simulink model "neuronchainv4"  (Simulink 7.6)
settings: Solver=ode45  StartTime=0.0  StopTime=10.0  RelTol=1e-3
values from neighbouring files (symbols this model uses):
  alpha = 0.8    [excneuroninit.m]
  beta = 0.05    [excneuroninit.m]
  inittime = 0.1    [excneuroninit.m]
  sigslopef = 1    [excneuroninit.m]
  sigslopei = 3    [excneuroninit.m]
  tau_s = 5    [excneuroninit.m]
libraries: simulink x480, neuronpoolibv3 x3
(part 1 of 17)
settings Model: Creator=root  LastModifiedBy=root

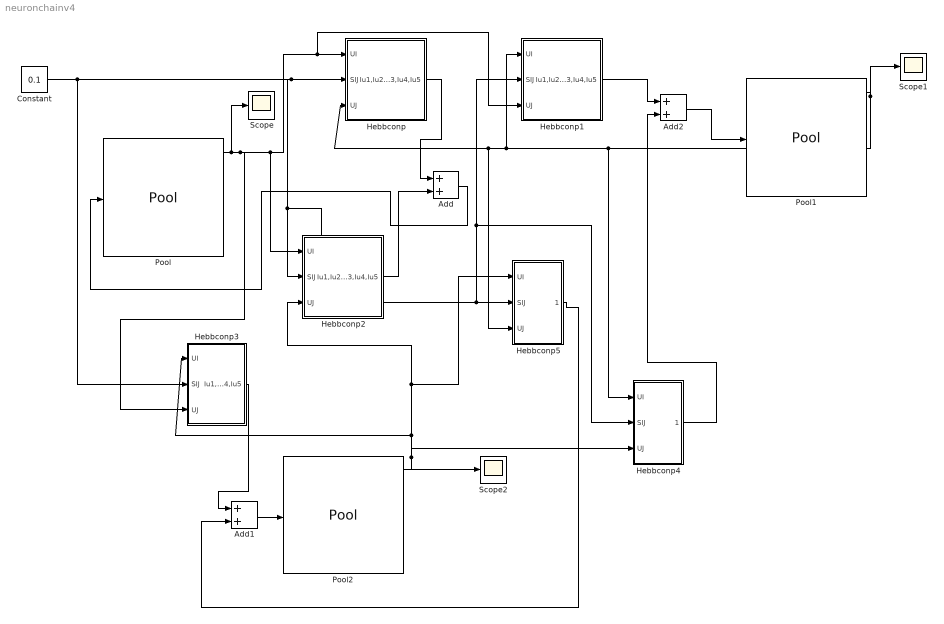
== system neuronchainv4 ==
  Add : Sum
  Add1 : Sum
  Add2 : Sum
  Constant : Constant  Value=0.1
  Hebbconp : Subsystem
  Hebbconp1 : Subsystem
  Hebbconp2 : Subsystem
  Hebbconp3 : Subsystem
  Hebbconp4 : Subsystem
  Hebbconp5 : Subsystem
  Pool : neuronpoolibv3/Pool  SystemSampleTime=-1
  Pool1 : neuronpoolibv3/Pool  SystemSampleTime=-1
  Pool2 : neuronpoolibv3/Pool  SystemSampleTime=-1
  Scope : Scope
  Scope1 : Scope
  Scope2 : Scope
      settings: SaveName=ScopeData2
  wires:
  Pool/1 -> Hebbconp/1(UI), Hebbconp1/3(UJ), Hebbconp2/1(UI), Hebbconp3/3(UJ), Scope/1
  Pool1/1 -> Hebbconp/3(UJ), Hebbconp5/3(UJ), Hebbconp1/1(UI), Hebbconp4/1(UI), Scope1/1
  Pool2/1 -> Hebbconp2/3(UJ), Hebbconp5/1(UI), Hebbconp3/1(UI), Scope2/1, Hebbconp4/3(UJ)
  Hebbconp2/1(Iu1,Iu2,Iu3,Iu4,Iu5) -> Add/2
  Hebbconp/1(Iu1,Iu2,Iu3,Iu4,Iu5) -> Add/1
  Add/1 -> Pool/1
  Hebbconp5/1(Iu1,Iu2,Iu3,Iu4,Iu5) -> Add1/2
  Hebbconp3/1(Iu1,Iu2,Iu3,Iu4,Iu5) -> Add1/1
  Add1/1 -> Pool2/1
  Hebbconp4/1(Iu1,Iu2,Iu3,Iu4,Iu5) -> Add2/2
  Hebbconp1/1(Iu1,Iu2,Iu3,Iu4,Iu5) -> Add2/1
  Add2/1 -> Pool1/1
  Constant/1 -> Hebbconp/2(SIJ), Hebbconp1/2(SIJ), Hebbconp4/2(SIJ), Hebbconp5/2(SIJ), Hebbconp2/2(SIJ), Hebbconp3/2(SIJ)

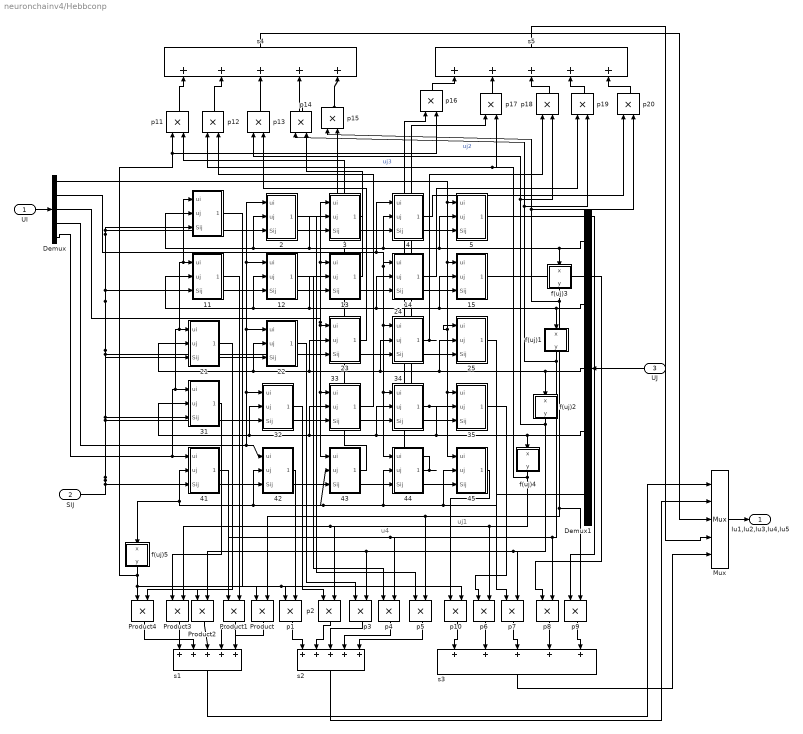
== system neuronchainv4/Hebbconp ==
  note: uj1
  note: u4
  UI : Inport
  SIJ : Inport  Port=2
  UJ : Inport  Port=3
  " " : Subsystem
  " 2" : Subsystem
  11 : Subsystem
  12 : Subsystem
  13 : Subsystem
  14 : Subsystem
  15 : Subsystem
  21 : Subsystem
  22 : Subsystem
  23 : Subsystem
  24 : Subsystem
  25 : Subsystem
  3 : Subsystem
  31 : Subsystem
  32 : Subsystem
  33 : Subsystem
  34 : Subsystem
  35 : Subsystem
  4 : Subsystem
  41 : Subsystem
  42 : Subsystem
  43 : Subsystem
  44 : Subsystem
  45 : Subsystem
  5 : Subsystem
  Demux : Demux  Outputs=5
  Demux1 : Demux  Outputs=5
  Mux : Mux  Inputs=5
  Product{,1..4} (5 alike) : Product  RndMeth=Zero
  f(uj)1 : Subsystem  TreatAsAtomicUnit=on  mask{slope=sigslopef, offset=0.5}
      mask help: Created by Han, Cheol
      mask Display: plot([10 15 20 25 30 35 40 45 50], [0 0.01 0.1 0.2 0.5 0.8 0.9 0.99 1])
  f(uj)2 : Subsystem  TreatAsAtomicUnit=on  mask{slope=sigslopef, offset=0.5}
      mask help: Created by Han, Cheol
      mask Display: plot([10 15 20 25 30 35 40 45 50], [0 0.01 0.1 0.2 0.5 0.8 0.9 0.99 1])
  f(uj)3 : Subsystem  TreatAsAtomicUnit=on  mask{slope=sigslopef, offset=0.5}
      mask help: Created by Han, Cheol
      mask Display: plot([10 15 20 25 30 35 40 45 50], [0 0.01 0.1 0.2 0.5 0.8 0.9 0.99 1])
  f(uj)4 : Subsystem  TreatAsAtomicUnit=on  mask{slope=sigslopef, offset=0.5}
      mask help: Created by Han, Cheol
      mask Display: plot([10 15 20 25 30 35 40 45 50], [0 0.01 0.1 0.2 0.5 0.8 0.9 0.99 1])
  f(uj)5 : Subsystem  TreatAsAtomicUnit=on  mask{slope=sigslopef, offset=0.5}
      mask help: Created by Han, Cheol
      mask Display: plot([10 15 20 25 30 35 40 45 50], [0 0.01 0.1 0.2 0.5 0.8 0.9 0.99 1])
  p{1..20} (20 alike) : Product  RndMeth=Zero
  s{1..5} (5 alike) : Sum  Inputs=+++++
  Iu1,Iu2,Iu3,Iu4,Iu5 : Outport
  wires:
  Demux/1 -> 15/1(ui), 45/1(ui), 35/1(ui), 25/1(ui), 5/1(ui)
  Demux/2 -> 4/1(ui), 44/1(ui), 34/1(ui), 24/1(ui), 14/1(ui)
  Demux/3 -> 43/1(ui), 33/1(ui), 23/1(ui), 13/1(ui), 3/1(ui)
  Demux/4 -> 42/1(ui), 32/1(ui), 22/1(ui), 12/1(ui), " 2"/1(ui)
  Demux/5 -> 41/1(ui), 31/1(ui), 21/1(ui), 11/1(ui), " "/1(ui)
  Demux1/1 -> " "/2(uj), " 2"/2(uj), 3/2(uj), 4/2(uj), 5/2(uj), f(uj)3/1(x)
  Demux1/2 -> 11/2(uj), 12/2(uj), 13/2(uj), 14/2(uj), 15/2(uj), f(uj)1/1(x)
  Demux1/3 -> 25/2(uj), 21/2(uj), 22/2(uj), 23/2(uj), 24/2(uj), f(uj)2/1(x)
  Demux1/4 -> 31/2(uj), 32/2(uj), 33/2(uj), 34/2(uj), 35/2(uj), f(uj)4/1(x)
  Demux1/5 -> 42/2(uj), 41/2(uj), f(uj)5/1(x), 43/2(uj), 44/2(uj), 45/2(uj)
  " "/1(Out1) -> Product/1
  11/1(Out1) -> Product1/2
  41/1(Out1) -> Product4/2
  21/1(Out1) -> Product2/1
  31/1(Out1) -> Product3/1
  f(uj)3/1(y) -> Product/2, p5/2, p9/2, p15/1, p20/2
  f(uj)1/1(y) -> Product1/1, p4/2, p8/2, p14/1, p19/2  "uj2"
  f(uj)2/1(y) -> Product2/2, p3/2, p7/2, p13/1, p18/2  "uj3"
  f(uj)4/1(y) -> Product3/2, p2/2, p6/2, p17/2, p12/1
  " 2"/1(Out1) -> p5/1
  12/1(Out1) -> p4/1
  22/1(Out1) -> p3/1
  32/1(Out1) -> p2/1
  42/1(Out1) -> p1/2
  f(uj)5/1(y) -> Product4/1, p1/1, p10/2, p11/1, p16/2
  5/1(Out1) -> p9/1
  15/1(Out1) -> p8/1
  25/1(Out1) -> p7/1
  35/1(Out1) -> p6/1
  45/1(Out1) -> p10/1
  3/1(Out1) -> p15/2
  13/1(Out1) -> p14/2
  23/1(Out1) -> p13/2
  33/1(Out1) -> p12/2
  43/1(Out1) -> p11/2
  p15/1 -> s4/5
  p11/1 -> s4/1
  p12/1 -> s4/2
  p13/1 -> s4/3
  p14/1 -> s4/4
  UI/1 -> Demux/1
  4/1(Out1) -> p20/1
  SIJ/1 -> 41/3(Sij), 21/3(Sij), 11/3(Sij), " "/3(Sij), " 2"/3(Sij), 3/3(Sij), 4/3(Sij), 5/3(Sij), 13/3(Sij), 14/3(Sij), 15/3(Sij), 12/3(Sij), 22/3(Sij), 23/3(Sij), 24/3(Sij), 25/3(Sij), 31/3(Sij), 33/3(Sij), 34/3(Sij), 35/3(Sij), 32/3(Sij), 42/3(Sij), 43/3(Sij), 44/3(Sij), 45/3(Sij)
  14/1(Out1) -> p19/1
  24/1(Out1) -> p18/1
  UJ/1 -> Demux1/1
  34/1(Out1) -> p17/1
  44/1(Out1) -> p16/1
  Product/1 -> s1/5
  Product1/1 -> s1/4
  Product2/1 -> s1/3
  Product3/1 -> s1/2
  Product4/1 -> s1/1
  p1/1 -> s2/1
  p10/1 -> s3/1
  p2/1 -> s2/2
  p3/1 -> s2/3
  p4/1 -> s2/4
  p5/1 -> s2/5
  p6/1 -> s3/2
  p7/1 -> s3/3
  p8/1 -> s3/4
  p9/1 -> s3/5
  p16/1 -> s5/1
  p17/1 -> s5/2
  p18/1 -> s5/3
  p19/1 -> s5/4
  p20/1 -> s5/5
  s4/1 -> Mux/3
  s1/1 -> Mux/1
  s2/1 -> Mux/2
  s3/1 -> Mux/5
  s5/1 -> Mux/4
  Mux/1 -> Iu1,Iu2,Iu3,Iu4,Iu5/1

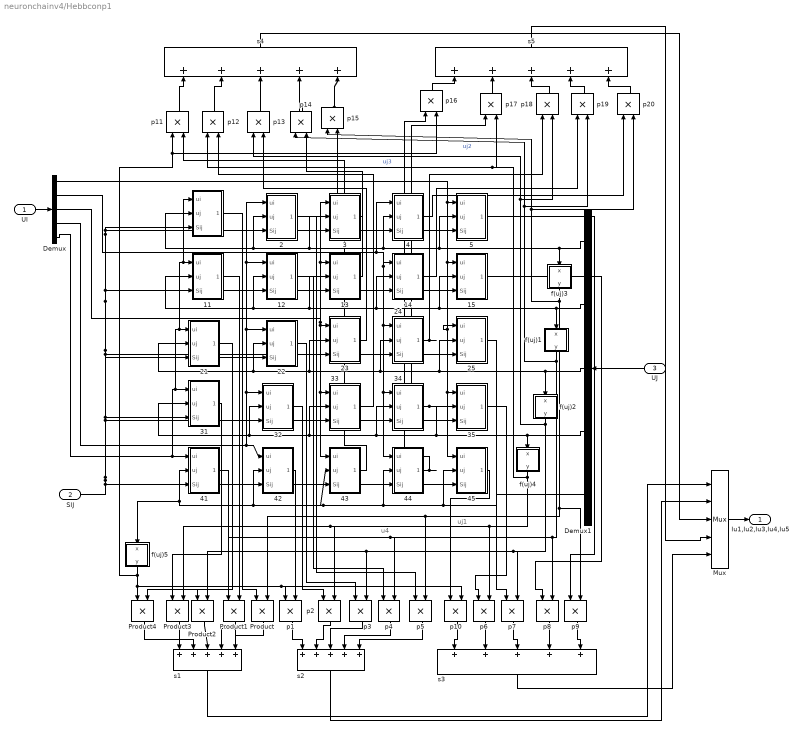
== system neuronchainv4/Hebbconp1 ==
  note: uj1
  note: u4
  UI : Inport
  SIJ : Inport  Port=2
  UJ : Inport  Port=3
  " " : Subsystem
  " 2" : Subsystem
  11 : Subsystem
  12 : Subsystem
  13 : Subsystem
  14 : Subsystem
  15 : Subsystem
  21 : Subsystem
  22 : Subsystem
  23 : Subsystem
  24 : Subsystem
  25 : Subsystem
  3 : Subsystem
  31 : Subsystem
  32 : Subsystem
  33 : Subsystem
  34 : Subsystem
  35 : Subsystem
  4 : Subsystem
  41 : Subsystem
  42 : Subsystem
  43 : Subsystem
  44 : Subsystem
  45 : Subsystem
  5 : Subsystem
  Demux : Demux  Outputs=5
  Demux1 : Demux  Outputs=5
  Mux : Mux  Inputs=5
  Product{,1..4} (5 alike) : Product  RndMeth=Zero
  f(uj)1 : Subsystem  TreatAsAtomicUnit=on  mask{slope=sigslopef, offset=0.5}
      mask help: Created by Han, Cheol
      mask Display: plot([10 15 20 25 30 35 40 45 50], [0 0.01 0.1 0.2 0.5 0.8 0.9 0.99 1])
  f(uj)2 : Subsystem  TreatAsAtomicUnit=on  mask{slope=sigslopef, offset=0.5}
      mask help: Created by Han, Cheol
      mask Display: plot([10 15 20 25 30 35 40 45 50], [0 0.01 0.1 0.2 0.5 0.8 0.9 0.99 1])
  f(uj)3 : Subsystem  TreatAsAtomicUnit=on  mask{slope=sigslopef, offset=0.5}
      mask help: Created by Han, Cheol
      mask Display: plot([10 15 20 25 30 35 40 45 50], [0 0.01 0.1 0.2 0.5 0.8 0.9 0.99 1])
  f(uj)4 : Subsystem  TreatAsAtomicUnit=on  mask{slope=sigslopef, offset=0.5}
      mask help: Created by Han, Cheol
      mask Display: plot([10 15 20 25 30 35 40 45 50], [0 0.01 0.1 0.2 0.5 0.8 0.9 0.99 1])
  f(uj)5 : Subsystem  TreatAsAtomicUnit=on  mask{slope=sigslopef, offset=0.5}
      mask help: Created by Han, Cheol
      mask Display: plot([10 15 20 25 30 35 40 45 50], [0 0.01 0.1 0.2 0.5 0.8 0.9 0.99 1])
  p{1..20} (20 alike) : Product  RndMeth=Zero
  s{1..5} (5 alike) : Sum  Inputs=+++++
  Iu1,Iu2,Iu3,Iu4,Iu5 : Outport
  wires:
  Demux/1 -> 15/1(ui), 45/1(ui), 35/1(ui), 25/1(ui), 5/1(ui)
  Demux/2 -> 4/1(ui), 44/1(ui), 34/1(ui), 24/1(ui), 14/1(ui)
  Demux/3 -> 43/1(ui), 33/1(ui), 23/1(ui), 13/1(ui), 3/1(ui)
  Demux/4 -> 42/1(ui), 32/1(ui), 22/1(ui), 12/1(ui), " 2"/1(ui)
  Demux/5 -> 41/1(ui), 31/1(ui), 21/1(ui), 11/1(ui), " "/1(ui)
  Demux1/1 -> " "/2(uj), " 2"/2(uj), 3/2(uj), 4/2(uj), 5/2(uj), f(uj)3/1(x)
  Demux1/2 -> 11/2(uj), 12/2(uj), 13/2(uj), 14/2(uj), 15/2(uj), f(uj)1/1(x)
  Demux1/3 -> 25/2(uj), 21/2(uj), 22/2(uj), 23/2(uj), 24/2(uj), f(uj)2/1(x)
  Demux1/4 -> 31/2(uj), 32/2(uj), 33/2(uj), 34/2(uj), 35/2(uj), f(uj)4/1(x)
  Demux1/5 -> 42/2(uj), 41/2(uj), f(uj)5/1(x), 43/2(uj), 44/2(uj), 45/2(uj)
  " "/1(Out1) -> Product/1
  11/1(Out1) -> Product1/2
  41/1(Out1) -> Product4/2
  21/1(Out1) -> Product2/1
  31/1(Out1) -> Product3/1
  f(uj)3/1(y) -> Product/2, p5/2, p9/2, p15/1, p20/2
  f(uj)1/1(y) -> Product1/1, p4/2, p8/2, p14/1, p19/2  "uj2"
  f(uj)2/1(y) -> Product2/2, p3/2, p7/2, p13/1, p18/2  "uj3"
  f(uj)4/1(y) -> Product3/2, p2/2, p6/2, p17/2, p12/1
  " 2"/1(Out1) -> p5/1
  12/1(Out1) -> p4/1
  22/1(Out1) -> p3/1
  32/1(Out1) -> p2/1
  42/1(Out1) -> p1/2
  f(uj)5/1(y) -> Product4/1, p1/1, p10/2, p11/1, p16/2
  5/1(Out1) -> p9/1
  15/1(Out1) -> p8/1
  25/1(Out1) -> p7/1
  35/1(Out1) -> p6/1
  45/1(Out1) -> p10/1
  3/1(Out1) -> p15/2
  13/1(Out1) -> p14/2
  23/1(Out1) -> p13/2
  33/1(Out1) -> p12/2
  43/1(Out1) -> p11/2
  p15/1 -> s4/5
  p11/1 -> s4/1
  p12/1 -> s4/2
  p13/1 -> s4/3
  p14/1 -> s4/4
  UI/1 -> Demux/1
  4/1(Out1) -> p20/1
  SIJ/1 -> 41/3(Sij), 21/3(Sij), 11/3(Sij), " "/3(Sij), " 2"/3(Sij), 3/3(Sij), 4/3(Sij), 5/3(Sij), 13/3(Sij), 14/3(Sij), 15/3(Sij), 12/3(Sij), 22/3(Sij), 23/3(Sij), 24/3(Sij), 25/3(Sij), 31/3(Sij), 33/3(Sij), 34/3(Sij), 35/3(Sij), 32/3(Sij), 42/3(Sij), 43/3(Sij), 44/3(Sij), 45/3(Sij)
  14/1(Out1) -> p19/1
  24/1(Out1) -> p18/1
  UJ/1 -> Demux1/1
  34/1(Out1) -> p17/1
  44/1(Out1) -> p16/1
  Product/1 -> s1/5
  Product1/1 -> s1/4
  Product2/1 -> s1/3
  Product3/1 -> s1/2
  Product4/1 -> s1/1
  p1/1 -> s2/1
  p10/1 -> s3/1
  p2/1 -> s2/2
  p3/1 -> s2/3
  p4/1 -> s2/4
  p5/1 -> s2/5
  p6/1 -> s3/2
  p7/1 -> s3/3
  p8/1 -> s3/4
  p9/1 -> s3/5
  p16/1 -> s5/1
  p17/1 -> s5/2
  p18/1 -> s5/3
  p19/1 -> s5/4
  p20/1 -> s5/5
  s4/1 -> Mux/3
  s1/1 -> Mux/1
  s2/1 -> Mux/2
  s3/1 -> Mux/5
  s5/1 -> Mux/4
  Mux/1 -> Iu1,Iu2,Iu3,Iu4,Iu5/1

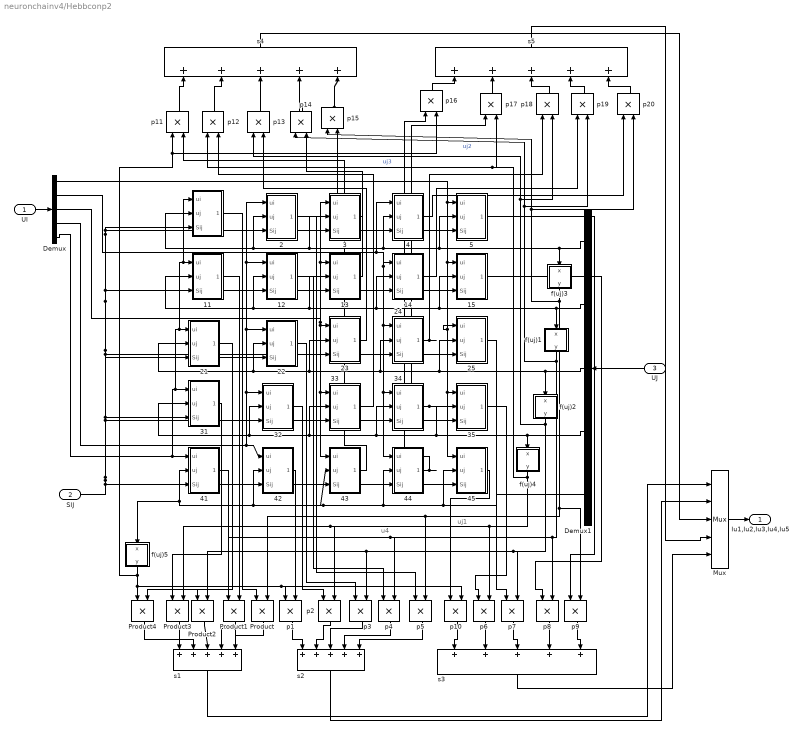
== system neuronchainv4/Hebbconp2 ==
  note: uj1
  note: u4
  UI : Inport
  SIJ : Inport  Port=2
  UJ : Inport  Port=3
  " " : Subsystem
  " 2" : Subsystem
  11 : Subsystem
  12 : Subsystem
  13 : Subsystem
  14 : Subsystem
  15 : Subsystem
  21 : Subsystem
  22 : Subsystem
  23 : Subsystem
  24 : Subsystem
  25 : Subsystem
  3 : Subsystem
  31 : Subsystem
  32 : Subsystem
  33 : Subsystem
  34 : Subsystem
  35 : Subsystem
  4 : Subsystem
  41 : Subsystem
  42 : Subsystem
  43 : Subsystem
  44 : Subsystem
  45 : Subsystem
  5 : Subsystem
  Demux : Demux  Outputs=5
  Demux1 : Demux  Outputs=5
  Mux : Mux  Inputs=5
  Product{,1..4} (5 alike) : Product  RndMeth=Zero
  f(uj)1 : Subsystem  TreatAsAtomicUnit=on  mask{slope=sigslopef, offset=0.5}
      mask help: Created by Han, Cheol
      mask Display: plot([10 15 20 25 30 35 40 45 50], [0 0.01 0.1 0.2 0.5 0.8 0.9 0.99 1])
  f(uj)2 : Subsystem  TreatAsAtomicUnit=on  mask{slope=sigslopef, offset=0.5}
      mask help: Created by Han, Cheol
      mask Display: plot([10 15 20 25 30 35 40 45 50], [0 0.01 0.1 0.2 0.5 0.8 0.9 0.99 1])
  f(uj)3 : Subsystem  TreatAsAtomicUnit=on  mask{slope=sigslopef, offset=0.5}
      mask help: Created by Han, Cheol
      mask Display: plot([10 15 20 25 30 35 40 45 50], [0 0.01 0.1 0.2 0.5 0.8 0.9 0.99 1])
  f(uj)4 : Subsystem  TreatAsAtomicUnit=on  mask{slope=sigslopef, offset=0.5}
      mask help: Created by Han, Cheol
      mask Display: plot([10 15 20 25 30 35 40 45 50], [0 0.01 0.1 0.2 0.5 0.8 0.9 0.99 1])
  f(uj)5 : Subsystem  TreatAsAtomicUnit=on  mask{slope=sigslopef, offset=0.5}
      mask help: Created by Han, Cheol
      mask Display: plot([10 15 20 25 30 35 40 45 50], [0 0.01 0.1 0.2 0.5 0.8 0.9 0.99 1])
  p{1..20} (20 alike) : Product  RndMeth=Zero
  s{1..5} (5 alike) : Sum  Inputs=+++++
  Iu1,Iu2,Iu3,Iu4,Iu5 : Outport
  wires:
  Demux/1 -> 15/1(ui), 45/1(ui), 35/1(ui), 25/1(ui), 5/1(ui)
  Demux/2 -> 4/1(ui), 44/1(ui), 34/1(ui), 24/1(ui), 14/1(ui)
  Demux/3 -> 43/1(ui), 33/1(ui), 23/1(ui), 13/1(ui), 3/1(ui)
  Demux/4 -> 42/1(ui), 32/1(ui), 22/1(ui), 12/1(ui), " 2"/1(ui)
  Demux/5 -> 41/1(ui), 31/1(ui), 21/1(ui), 11/1(ui), " "/1(ui)
  Demux1/1 -> " "/2(uj), " 2"/2(uj), 3/2(uj), 4/2(uj), 5/2(uj), f(uj)3/1(x)
  Demux1/2 -> 11/2(uj), 12/2(uj), 13/2(uj), 14/2(uj), 15/2(uj), f(uj)1/1(x)
  Demux1/3 -> 25/2(uj), 21/2(uj), 22/2(uj), 23/2(uj), 24/2(uj), f(uj)2/1(x)
  Demux1/4 -> 31/2(uj), 32/2(uj), 33/2(uj), 34/2(uj), 35/2(uj), f(uj)4/1(x)
  Demux1/5 -> 42/2(uj), 41/2(uj), f(uj)5/1(x), 43/2(uj), 44/2(uj), 45/2(uj)
  " "/1(Out1) -> Product/1
  11/1(Out1) -> Product1/2
  41/1(Out1) -> Product4/2
  21/1(Out1) -> Product2/1
  31/1(Out1) -> Product3/1
  f(uj)3/1(y) -> Product/2, p5/2, p9/2, p15/1, p20/2
  f(uj)1/1(y) -> Product1/1, p4/2, p8/2, p14/1, p19/2  "uj2"
  f(uj)2/1(y) -> Product2/2, p3/2, p7/2, p13/1, p18/2  "uj3"
  f(uj)4/1(y) -> Product3/2, p2/2, p6/2, p17/2, p12/1
  " 2"/1(Out1) -> p5/1
  12/1(Out1) -> p4/1
  22/1(Out1) -> p3/1
  32/1(Out1) -> p2/1
  42/1(Out1) -> p1/2
  f(uj)5/1(y) -> Product4/1, p1/1, p10/2, p11/1, p16/2
  5/1(Out1) -> p9/1
  15/1(Out1) -> p8/1
  25/1(Out1) -> p7/1
  35/1(Out1) -> p6/1
  45/1(Out1) -> p10/1
  3/1(Out1) -> p15/2
  13/1(Out1) -> p14/2
  23/1(Out1) -> p13/2
  33/1(Out1) -> p12/2
  43/1(Out1) -> p11/2
  p15/1 -> s4/5
  p11/1 -> s4/1
  p12/1 -> s4/2
  p13/1 -> s4/3
  p14/1 -> s4/4
  UI/1 -> Demux/1
  4/1(Out1) -> p20/1
  SIJ/1 -> 41/3(Sij), 21/3(Sij), 11/3(Sij), " "/3(Sij), " 2"/3(Sij), 3/3(Sij), 4/3(Sij), 5/3(Sij), 13/3(Sij), 14/3(Sij), 15/3(Sij), 12/3(Sij), 22/3(Sij), 23/3(Sij), 24/3(Sij), 25/3(Sij), 31/3(Sij), 33/3(Sij), 34/3(Sij), 35/3(Sij), 32/3(Sij), 42/3(Sij), 43/3(Sij), 44/3(Sij), 45/3(Sij)
  14/1(Out1) -> p19/1
  24/1(Out1) -> p18/1
  UJ/1 -> Demux1/1
  34/1(Out1) -> p17/1
  44/1(Out1) -> p16/1
  Product/1 -> s1/5
  Product1/1 -> s1/4
  Product2/1 -> s1/3
  Product3/1 -> s1/2
  Product4/1 -> s1/1
  p1/1 -> s2/1
  p10/1 -> s3/1
  p2/1 -> s2/2
  p3/1 -> s2/3
  p4/1 -> s2/4
  p5/1 -> s2/5
  p6/1 -> s3/2
  p7/1 -> s3/3
  p8/1 -> s3/4
  p9/1 -> s3/5
  p16/1 -> s5/1
  p17/1 -> s5/2
  p18/1 -> s5/3
  p19/1 -> s5/4
  p20/1 -> s5/5
  s4/1 -> Mux/3
  s1/1 -> Mux/1
  s2/1 -> Mux/2
  s3/1 -> Mux/5
  s5/1 -> Mux/4
  Mux/1 -> Iu1,Iu2,Iu3,Iu4,Iu5/1

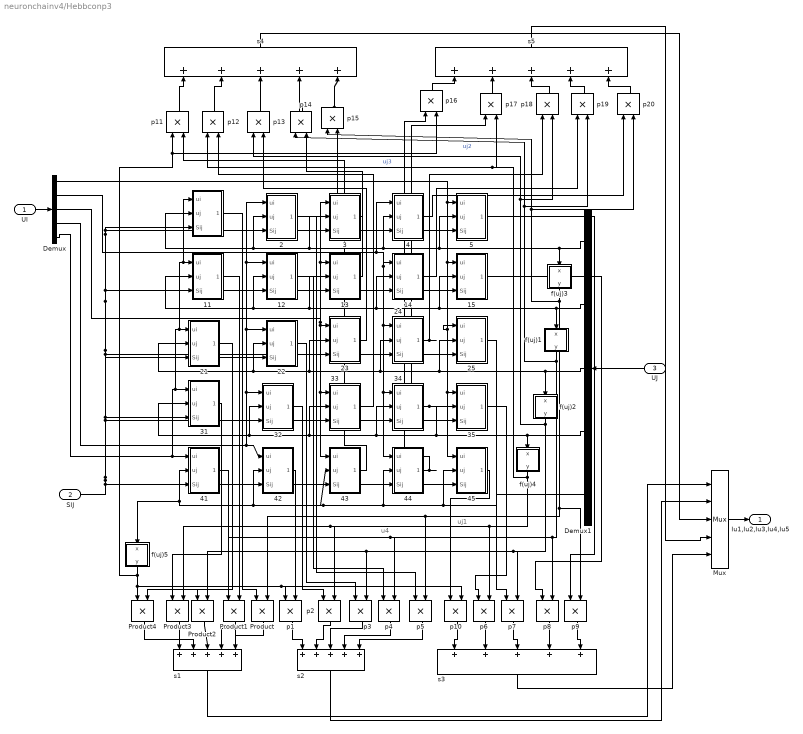
== system neuronchainv4/Hebbconp3 ==
  note: uj1
  note: u4
  UI : Inport
  SIJ : Inport  Port=2
  UJ : Inport  Port=3
  " " : Subsystem
  " 2" : Subsystem
  11 : Subsystem
  12 : Subsystem
  13 : Subsystem
  14 : Subsystem
  15 : Subsystem
  21 : Subsystem
  22 : Subsystem
  23 : Subsystem
  24 : Subsystem
  25 : Subsystem
  3 : Subsystem
  31 : Subsystem
  32 : Subsystem
  33 : Subsystem
  34 : Subsystem
  35 : Subsystem
  4 : Subsystem
  41 : Subsystem
  42 : Subsystem
  43 : Subsystem
  44 : Subsystem
  45 : Subsystem
  5 : Subsystem
  Demux : Demux  Outputs=5
  Demux1 : Demux  Outputs=5
  Mux : Mux  Inputs=5
  Product{,1..4} (5 alike) : Product  RndMeth=Zero
  f(uj)1 : Subsystem  TreatAsAtomicUnit=on  mask{slope=sigslopef, offset=0.5}
      mask help: Created by Han, Cheol
      mask Display: plot([10 15 20 25 30 35 40 45 50], [0 0.01 0.1 0.2 0.5 0.8 0.9 0.99 1])
  f(uj)2 : Subsystem  TreatAsAtomicUnit=on  mask{slope=sigslopef, offset=0.5}
      mask help: Created by Han, Cheol
      mask Display: plot([10 15 20 25 30 35 40 45 50], [0 0.01 0.1 0.2 0.5 0.8 0.9 0.99 1])
  f(uj)3 : Subsystem  TreatAsAtomicUnit=on  mask{slope=sigslopef, offset=0.5}
      mask help: Created by Han, Cheol
      mask Display: plot([10 15 20 25 30 35 40 45 50], [0 0.01 0.1 0.2 0.5 0.8 0.9 0.99 1])
  f(uj)4 : Subsystem  TreatAsAtomicUnit=on  mask{slope=sigslopef, offset=0.5}
      mask help: Created by Han, Cheol
      mask Display: plot([10 15 20 25 30 35 40 45 50], [0 0.01 0.1 0.2 0.5 0.8 0.9 0.99 1])
  f(uj)5 : Subsystem  TreatAsAtomicUnit=on  mask{slope=sigslopef, offset=0.5}
      mask help: Created by Han, Cheol
      mask Display: plot([10 15 20 25 30 35 40 45 50], [0 0.01 0.1 0.2 0.5 0.8 0.9 0.99 1])
  p{1..20} (20 alike) : Product  RndMeth=Zero
  s{1..5} (5 alike) : Sum  Inputs=+++++
  Iu1,Iu2,Iu3,Iu4,Iu5 : Outport
  wires:
  Demux/1 -> 15/1(ui), 45/1(ui), 35/1(ui), 25/1(ui), 5/1(ui)
  Demux/2 -> 4/1(ui), 44/1(ui), 34/1(ui), 24/1(ui), 14/1(ui)
  Demux/3 -> 43/1(ui), 33/1(ui), 23/1(ui), 13/1(ui), 3/1(ui)
  Demux/4 -> 42/1(ui), 32/1(ui), 22/1(ui), 12/1(ui), " 2"/1(ui)
  Demux/5 -> 41/1(ui), 31/1(ui), 21/1(ui), 11/1(ui), " "/1(ui)
  Demux1/1 -> " "/2(uj), " 2"/2(uj), 3/2(uj), 4/2(uj), 5/2(uj), f(uj)3/1(x)
  Demux1/2 -> 11/2(uj), 12/2(uj), 13/2(uj), 14/2(uj), 15/2(uj), f(uj)1/1(x)
  Demux1/3 -> 25/2(uj), 21/2(uj), 22/2(uj), 23/2(uj), 24/2(uj), f(uj)2/1(x)
  Demux1/4 -> 31/2(uj), 32/2(uj), 33/2(uj), 34/2(uj), 35/2(uj), f(uj)4/1(x)
  Demux1/5 -> 42/2(uj), 41/2(uj), f(uj)5/1(x), 43/2(uj), 44/2(uj), 45/2(uj)
  " "/1(Out1) -> Product/1
  11/1(Out1) -> Product1/2
  41/1(Out1) -> Product4/2
  21/1(Out1) -> Product2/1
  31/1(Out1) -> Product3/1
  f(uj)3/1(y) -> Product/2, p5/2, p9/2, p15/1, p20/2
  f(uj)1/1(y) -> Product1/1, p4/2, p8/2, p14/1, p19/2  "uj2"
  f(uj)2/1(y) -> Product2/2, p3/2, p7/2, p13/1, p18/2  "uj3"
  f(uj)4/1(y) -> Product3/2, p2/2, p6/2, p17/2, p12/1
  " 2"/1(Out1) -> p5/1
  12/1(Out1) -> p4/1
  22/1(Out1) -> p3/1
  32/1(Out1) -> p2/1
  42/1(Out1) -> p1/2
  f(uj)5/1(y) -> Product4/1, p1/1, p10/2, p11/1, p16/2
  5/1(Out1) -> p9/1
  15/1(Out1) -> p8/1
  25/1(Out1) -> p7/1
  35/1(Out1) -> p6/1
  45/1(Out1) -> p10/1
  3/1(Out1) -> p15/2
  13/1(Out1) -> p14/2
  23/1(Out1) -> p13/2
  33/1(Out1) -> p12/2
  43/1(Out1) -> p11/2
  p15/1 -> s4/5
  p11/1 -> s4/1
  p12/1 -> s4/2
  p13/1 -> s4/3
  p14/1 -> s4/4
  UI/1 -> Demux/1
  4/1(Out1) -> p20/1
  SIJ/1 -> 41/3(Sij), 21/3(Sij), 11/3(Sij), " "/3(Sij), " 2"/3(Sij), 3/3(Sij), 4/3(Sij), 5/3(Sij), 13/3(Sij), 14/3(Sij), 15/3(Sij), 12/3(Sij), 22/3(Sij), 23/3(Sij), 24/3(Sij), 25/3(Sij), 31/3(Sij), 33/3(Sij), 34/3(Sij), 35/3(Sij), 32/3(Sij), 42/3(Sij), 43/3(Sij), 44/3(Sij), 45/3(Sij)
  14/1(Out1) -> p19/1
  24/1(Out1) -> p18/1
  UJ/1 -> Demux1/1
  34/1(Out1) -> p17/1
  44/1(Out1) -> p16/1
  Product/1 -> s1/5
  Product1/1 -> s1/4
  Product2/1 -> s1/3
  Product3/1 -> s1/2
  Product4/1 -> s1/1
  p1/1 -> s2/1
  p10/1 -> s3/1
  p2/1 -> s2/2
  p3/1 -> s2/3
  p4/1 -> s2/4
  p5/1 -> s2/5
  p6/1 -> s3/2
  p7/1 -> s3/3
  p8/1 -> s3/4
  p9/1 -> s3/5
  p16/1 -> s5/1
  p17/1 -> s5/2
  p18/1 -> s5/3
  p19/1 -> s5/4
  p20/1 -> s5/5
  s4/1 -> Mux/3
  s1/1 -> Mux/1
  s2/1 -> Mux/2
  s3/1 -> Mux/5
  s5/1 -> Mux/4
  Mux/1 -> Iu1,Iu2,Iu3,Iu4,Iu5/1

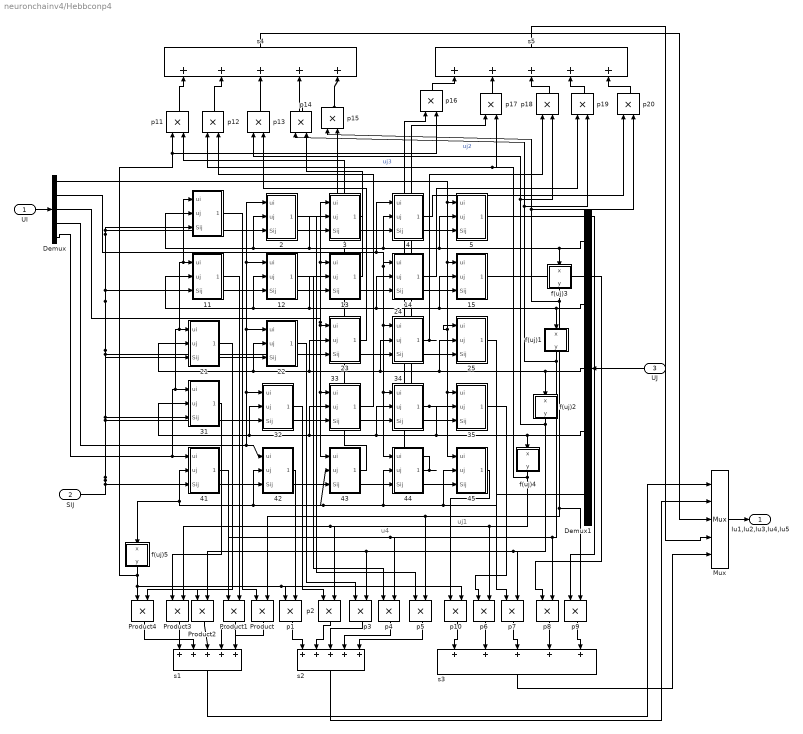
== system neuronchainv4/Hebbconp4 ==
  note: uj1
  note: u4
  UI : Inport
  SIJ : Inport  Port=2
  UJ : Inport  Port=3
  " " : Subsystem
  " 2" : Subsystem
  11 : Subsystem
  12 : Subsystem
  13 : Subsystem
  14 : Subsystem
  15 : Subsystem
  21 : Subsystem
  22 : Subsystem
  23 : Subsystem
  24 : Subsystem
  25 : Subsystem
  3 : Subsystem
  31 : Subsystem
  32 : Subsystem
  33 : Subsystem
  34 : Subsystem
  35 : Subsystem
  4 : Subsystem
  41 : Subsystem
  42 : Subsystem
  43 : Subsystem
  44 : Subsystem
  45 : Subsystem
  5 : Subsystem
  Demux : Demux  Outputs=5
  Demux1 : Demux  Outputs=5
  Mux : Mux  Inputs=5
  Product{,1..4} (5 alike) : Product  RndMeth=Zero
  f(uj)1 : Subsystem  TreatAsAtomicUnit=on  mask{slope=sigslopef, offset=0.5}
      mask help: Created by Han, Cheol
      mask Display: plot([10 15 20 25 30 35 40 45 50], [0 0.01 0.1 0.2 0.5 0.8 0.9 0.99 1])
  f(uj)2 : Subsystem  TreatAsAtomicUnit=on  mask{slope=sigslopef, offset=0.5}
      mask help: Created by Han, Cheol
      mask Display: plot([10 15 20 25 30 35 40 45 50], [0 0.01 0.1 0.2 0.5 0.8 0.9 0.99 1])
  f(uj)3 : Subsystem  TreatAsAtomicUnit=on  mask{slope=sigslopef, offset=0.5}
      mask help: Created by Han, Cheol
      mask Display: plot([10 15 20 25 30 35 40 45 50], [0 0.01 0.1 0.2 0.5 0.8 0.9 0.99 1])
  f(uj)4 : Subsystem  TreatAsAtomicUnit=on  mask{slope=sigslopef, offset=0.5}
      mask help: Created by Han, Cheol
      mask Display: plot([10 15 20 25 30 35 40 45 50], [0 0.01 0.1 0.2 0.5 0.8 0.9 0.99 1])
  f(uj)5 : Subsystem  TreatAsAtomicUnit=on  mask{slope=sigslopef, offset=0.5}
      mask help: Created by Han, Cheol
      mask Display: plot([10 15 20 25 30 35 40 45 50], [0 0.01 0.1 0.2 0.5 0.8 0.9 0.99 1])
  p{1..20} (20 alike) : Product  RndMeth=Zero
  s{1..5} (5 alike) : Sum  Inputs=+++++
  Iu1,Iu2,Iu3,Iu4,Iu5 : Outport
  wires:
  Demux/1 -> 15/1(ui), 45/1(ui), 35/1(ui), 25/1(ui), 5/1(ui)
  Demux/2 -> 4/1(ui), 44/1(ui), 34/1(ui), 24/1(ui), 14/1(ui)
  Demux/3 -> 43/1(ui), 33/1(ui), 23/1(ui), 13/1(ui), 3/1(ui)
  Demux/4 -> 42/1(ui), 32/1(ui), 22/1(ui), 12/1(ui), " 2"/1(ui)
  Demux/5 -> 41/1(ui), 31/1(ui), 21/1(ui), 11/1(ui), " "/1(ui)
  Demux1/1 -> " "/2(uj), " 2"/2(uj), 3/2(uj), 4/2(uj), 5/2(uj), f(uj)3/1(x)
  Demux1/2 -> 11/2(uj), 12/2(uj), 13/2(uj), 14/2(uj), 15/2(uj), f(uj)1/1(x)
  Demux1/3 -> 25/2(uj), 21/2(uj), 22/2(uj), 23/2(uj), 24/2(uj), f(uj)2/1(x)
  Demux1/4 -> 31/2(uj), 32/2(uj), 33/2(uj), 34/2(uj), 35/2(uj), f(uj)4/1(x)
  Demux1/5 -> 42/2(uj), 41/2(uj), f(uj)5/1(x), 43/2(uj), 44/2(uj), 45/2(uj)
  " "/1(Out1) -> Product/1
  11/1(Out1) -> Product1/2
  41/1(Out1) -> Product4/2
  21/1(Out1) -> Product2/1
  31/1(Out1) -> Product3/1
  f(uj)3/1(y) -> Product/2, p5/2, p9/2, p15/1, p20/2
  f(uj)1/1(y) -> Product1/1, p4/2, p8/2, p14/1, p19/2  "uj2"
  f(uj)2/1(y) -> Product2/2, p3/2, p7/2, p13/1, p18/2  "uj3"
  f(uj)4/1(y) -> Product3/2, p2/2, p6/2, p17/2, p12/1
  " 2"/1(Out1) -> p5/1
  12/1(Out1) -> p4/1
  22/1(Out1) -> p3/1
  32/1(Out1) -> p2/1
  42/1(Out1) -> p1/2
  f(uj)5/1(y) -> Product4/1, p1/1, p10/2, p11/1, p16/2
  5/1(Out1) -> p9/1
  15/1(Out1) -> p8/1
  25/1(Out1) -> p7/1
  35/1(Out1) -> p6/1
  45/1(Out1) -> p10/1
  3/1(Out1) -> p15/2
  13/1(Out1) -> p14/2
  23/1(Out1) -> p13/2
  33/1(Out1) -> p12/2
  43/1(Out1) -> p11/2
  p15/1 -> s4/5
  p11/1 -> s4/1
  p12/1 -> s4/2
  p13/1 -> s4/3
  p14/1 -> s4/4
  UI/1 -> Demux/1
  4/1(Out1) -> p20/1
  SIJ/1 -> 41/3(Sij), 21/3(Sij), 11/3(Sij), " "/3(Sij), " 2"/3(Sij), 3/3(Sij), 4/3(Sij), 5/3(Sij), 13/3(Sij), 14/3(Sij), 15/3(Sij), 12/3(Sij), 22/3(Sij), 23/3(Sij), 24/3(Sij), 25/3(Sij), 31/3(Sij), 33/3(Sij), 34/3(Sij), 35/3(Sij), 32/3(Sij), 42/3(Sij), 43/3(Sij), 44/3(Sij), 45/3(Sij)
  14/1(Out1) -> p19/1
  24/1(Out1) -> p18/1
  UJ/1 -> Demux1/1
  34/1(Out1) -> p17/1
  44/1(Out1) -> p16/1
  Product/1 -> s1/5
  Product1/1 -> s1/4
  Product2/1 -> s1/3
  Product3/1 -> s1/2
  Product4/1 -> s1/1
  p1/1 -> s2/1
  p10/1 -> s3/1
  p2/1 -> s2/2
  p3/1 -> s2/3
  p4/1 -> s2/4
  p5/1 -> s2/5
  p6/1 -> s3/2
  p7/1 -> s3/3
  p8/1 -> s3/4
  p9/1 -> s3/5
  p16/1 -> s5/1
  p17/1 -> s5/2
  p18/1 -> s5/3
  p19/1 -> s5/4
  p20/1 -> s5/5
  s4/1 -> Mux/3
  s1/1 -> Mux/1
  s2/1 -> Mux/2
  s3/1 -> Mux/5
  s5/1 -> Mux/4
  Mux/1 -> Iu1,Iu2,Iu3,Iu4,Iu5/1

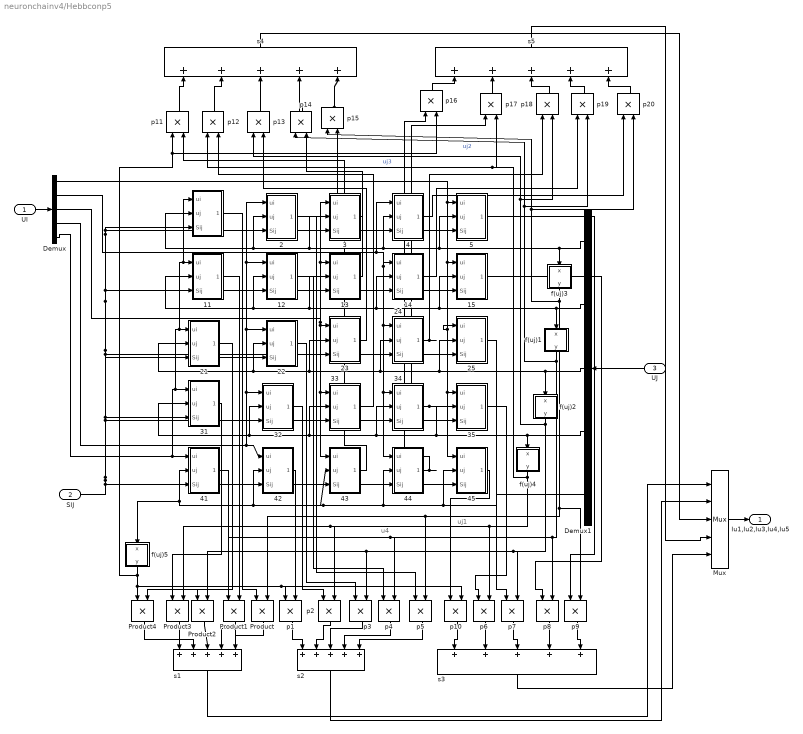
== system neuronchainv4/Hebbconp5 ==
  note: uj1
  note: u4
  UI : Inport
  SIJ : Inport  Port=2
  UJ : Inport  Port=3
  " " : Subsystem
  " 2" : Subsystem
  11 : Subsystem
  12 : Subsystem
  13 : Subsystem
  14 : Subsystem
  15 : Subsystem
  21 : Subsystem
  22 : Subsystem
  23 : Subsystem
  24 : Subsystem
  25 : Subsystem
  3 : Subsystem
  31 : Subsystem
  32 : Subsystem
  33 : Subsystem
  34 : Subsystem
  35 : Subsystem
  4 : Subsystem
  41 : Subsystem
  42 : Subsystem
  43 : Subsystem
  44 : Subsystem
  45 : Subsystem
  5 : Subsystem
  Demux : Demux  Outputs=5
  Demux1 : Demux  Outputs=5
  Mux : Mux  Inputs=5
  Product{,1..4} (5 alike) : Product  RndMeth=Zero
  f(uj)1 : Subsystem  TreatAsAtomicUnit=on  mask{slope=sigslopef, offset=0.5}
      mask help: Created by Han, Cheol
      mask Display: plot([10 15 20 25 30 35 40 45 50], [0 0.01 0.1 0.2 0.5 0.8 0.9 0.99 1])
  f(uj)2 : Subsystem  TreatAsAtomicUnit=on  mask{slope=sigslopef, offset=0.5}
      mask help: Created by Han, Cheol
      mask Display: plot([10 15 20 25 30 35 40 45 50], [0 0.01 0.1 0.2 0.5 0.8 0.9 0.99 1])
  f(uj)3 : Subsystem  TreatAsAtomicUnit=on  mask{slope=sigslopef, offset=0.5}
      mask help: Created by Han, Cheol
      mask Display: plot([10 15 20 25 30 35 40 45 50], [0 0.01 0.1 0.2 0.5 0.8 0.9 0.99 1])
  f(uj)4 : Subsystem  TreatAsAtomicUnit=on  mask{slope=sigslopef, offset=0.5}
      mask help: Created by Han, Cheol
      mask Display: plot([10 15 20 25 30 35 40 45 50], [0 0.01 0.1 0.2 0.5 0.8 0.9 0.99 1])
  f(uj)5 : Subsystem  TreatAsAtomicUnit=on  mask{slope=sigslopef, offset=0.5}
      mask help: Created by Han, Cheol
      mask Display: plot([10 15 20 25 30 35 40 45 50], [0 0.01 0.1 0.2 0.5 0.8 0.9 0.99 1])
  p{1..20} (20 alike) : Product  RndMeth=Zero
  s{1..5} (5 alike) : Sum  Inputs=+++++
  Iu1,Iu2,Iu3,Iu4,Iu5 : Outport
  wires:
  Demux/1 -> 15/1(ui), 45/1(ui), 35/1(ui), 25/1(ui), 5/1(ui)
  Demux/2 -> 4/1(ui), 44/1(ui), 34/1(ui), 24/1(ui), 14/1(ui)
  Demux/3 -> 43/1(ui), 33/1(ui), 23/1(ui), 13/1(ui), 3/1(ui)
  Demux/4 -> 42/1(ui), 32/1(ui), 22/1(ui), 12/1(ui), " 2"/1(ui)
  Demux/5 -> 41/1(ui), 31/1(ui), 21/1(ui), 11/1(ui), " "/1(ui)
  Demux1/1 -> " "/2(uj), " 2"/2(uj), 3/2(uj), 4/2(uj), 5/2(uj), f(uj)3/1(x)
  Demux1/2 -> 11/2(uj), 12/2(uj), 13/2(uj), 14/2(uj), 15/2(uj), f(uj)1/1(x)
  Demux1/3 -> 25/2(uj), 21/2(uj), 22/2(uj), 23/2(uj), 24/2(uj), f(uj)2/1(x)
  Demux1/4 -> 31/2(uj), 32/2(uj), 33/2(uj), 34/2(uj), 35/2(uj), f(uj)4/1(x)
  Demux1/5 -> 42/2(uj), 41/2(uj), f(uj)5/1(x), 43/2(uj), 44/2(uj), 45/2(uj)
  " "/1(Out1) -> Product/1
  11/1(Out1) -> Product1/2
  41/1(Out1) -> Product4/2
  21/1(Out1) -> Product2/1
  31/1(Out1) -> Product3/1
  f(uj)3/1(y) -> Product/2, p5/2, p9/2, p15/1, p20/2
  f(uj)1/1(y) -> Product1/1, p4/2, p8/2, p14/1, p19/2  "uj2"
  f(uj)2/1(y) -> Product2/2, p3/2, p7/2, p13/1, p18/2  "uj3"
  f(uj)4/1(y) -> Product3/2, p2/2, p6/2, p17/2, p12/1
  " 2"/1(Out1) -> p5/1
  12/1(Out1) -> p4/1
  22/1(Out1) -> p3/1
  32/1(Out1) -> p2/1
  42/1(Out1) -> p1/2
  f(uj)5/1(y) -> Product4/1, p1/1, p10/2, p11/1, p16/2
  5/1(Out1) -> p9/1
  15/1(Out1) -> p8/1
  25/1(Out1) -> p7/1
  35/1(Out1) -> p6/1
  45/1(Out1) -> p10/1
  3/1(Out1) -> p15/2
  13/1(Out1) -> p14/2
  23/1(Out1) -> p13/2
  33/1(Out1) -> p12/2
  43/1(Out1) -> p11/2
  p15/1 -> s4/5
  p11/1 -> s4/1
  p12/1 -> s4/2
  p13/1 -> s4/3
  p14/1 -> s4/4
  UI/1 -> Demux/1
  4/1(Out1) -> p20/1
  SIJ/1 -> 41/3(Sij), 21/3(Sij), 11/3(Sij), " "/3(Sij), " 2"/3(Sij), 3/3(Sij), 4/3(Sij), 5/3(Sij), 13/3(Sij), 14/3(Sij), 15/3(Sij), 12/3(Sij), 22/3(Sij), 23/3(Sij), 24/3(Sij), 25/3(Sij), 31/3(Sij), 33/3(Sij), 34/3(Sij), 35/3(Sij), 32/3(Sij), 42/3(Sij), 43/3(Sij), 44/3(Sij), 45/3(Sij)
  14/1(Out1) -> p19/1
  24/1(Out1) -> p18/1
  UJ/1 -> Demux1/1
  34/1(Out1) -> p17/1
  44/1(Out1) -> p16/1
  Product/1 -> s1/5
  Product1/1 -> s1/4
  Product2/1 -> s1/3
  Product3/1 -> s1/2
  Product4/1 -> s1/1
  p1/1 -> s2/1
  p10/1 -> s3/1
  p2/1 -> s2/2
  p3/1 -> s2/3
  p4/1 -> s2/4
  p5/1 -> s2/5
  p6/1 -> s3/2
  p7/1 -> s3/3
  p8/1 -> s3/4
  p9/1 -> s3/5
  p16/1 -> s5/1
  p17/1 -> s5/2
  p18/1 -> s5/3
  p19/1 -> s5/4
  p20/1 -> s5/5
  s4/1 -> Mux/3
  s1/1 -> Mux/1
  s2/1 -> Mux/2
  s3/1 -> Mux/5
  s5/1 -> Mux/4
  Mux/1 -> Iu1,Iu2,Iu3,Iu4,Iu5/1

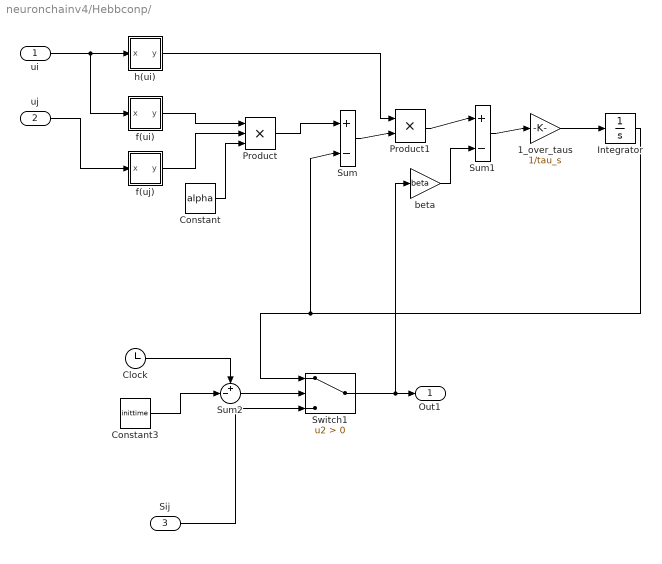
== system neuronchainv4/Hebbconp/  ==
  ui : Inport
  uj : Inport  Port=2
  Sij : Inport  Port=3
  1_over_taus : Gain  Gain=1/tau_s
  Clock : Clock
      settings: Decimation=10
  Constant : Constant  Value=alpha
  Constant3 : Constant  Value=inittime
  Integrator : Integrator
  Product : Product  Inputs=3  RndMeth=Zero
  Product1 : Product  RndMeth=Zero
  Sum : Sum  Inputs=|+-
  Sum1 : Sum  Inputs=|+-
  Sum2 : Sum  Inputs=+-|
  Switch1 : Switch  Criteria=u2 > Threshold
  beta : Gain  Gain=beta
  f(ui) : Subsystem  TreatAsAtomicUnit=on  mask{slope=sigslopef, offset=0.5}
      mask help: Created by Han, Cheol
      mask Display: plot([10 15 20 25 30 35 40 45 50], [0 0.01 0.1 0.2 0.5 0.8 0.9 0.99 1])
  f(uj) : Subsystem  TreatAsAtomicUnit=on  mask{slope=sigslopef, offset=0.5}
      mask help: Created by Han, Cheol
      mask Display: plot([10 15 20 25 30 35 40 45 50], [0 0.01 0.1 0.2 0.5 0.8 0.9 0.99 1])
  h(ui) : Subsystem  TreatAsAtomicUnit=on  mask{slope=sigslopei, offset=0.5}
      mask help: Created by Han, Cheol
      mask Display: plot([10 15 20 25 30 35 40 45 50], [0 0.01 0.1 0.2 0.5 0.8 0.9 0.99 1])
  Out1 : Outport
  wires:
  ui/1 -> h(ui)/1(x), f(ui)/1(x)
  uj/1 -> f(uj)/1(x)
  f(ui)/1(y) -> Product/1
  f(uj)/1(y) -> Product/2
  Constant/1 -> Product/3
  Product/1 -> Sum/1
  Sum/1 -> Product1/2
  h(ui)/1(y) -> Product1/1
  Product1/1 -> Sum1/1
  beta/1 -> Sum1/2
  Sum1/1 -> 1_over_taus/1
  1_over_taus/1 -> Integrator/1
  Integrator/1 -> Switch1/1, Sum/2
  Sum2/1 -> Switch1/2
  Clock/1 -> Sum2/1
  Constant3/1 -> Sum2/2
  Switch1/1 -> beta/1, Out1/1
  Sij/1 -> Switch1/3

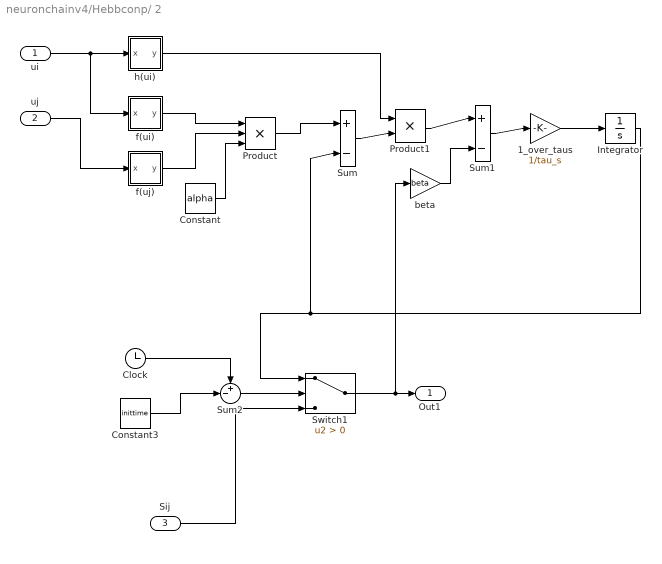
== system neuronchainv4/Hebbconp/ 2 ==
  ui : Inport
  uj : Inport  Port=2
  Sij : Inport  Port=3
  1_over_taus : Gain  Gain=1/tau_s
  Clock : Clock
      settings: Decimation=10
  Constant : Constant  Value=alpha
  Constant3 : Constant  Value=inittime
  Integrator : Integrator
  Product : Product  Inputs=3  RndMeth=Zero
  Product1 : Product  RndMeth=Zero
  Sum : Sum  Inputs=|+-
  Sum1 : Sum  Inputs=|+-
  Sum2 : Sum  Inputs=+-|
  Switch1 : Switch  Criteria=u2 > Threshold
  beta : Gain  Gain=beta
  f(ui) : Subsystem  TreatAsAtomicUnit=on  mask{slope=sigslopef, offset=0.5}
      mask help: Created by Han, Cheol
      mask Display: plot([10 15 20 25 30 35 40 45 50], [0 0.01 0.1 0.2 0.5 0.8 0.9 0.99 1])
  f(uj) : Subsystem  TreatAsAtomicUnit=on  mask{slope=sigslopef, offset=0.5}
      mask help: Created by Han, Cheol
      mask Display: plot([10 15 20 25 30 35 40 45 50], [0 0.01 0.1 0.2 0.5 0.8 0.9 0.99 1])
  h(ui) : Subsystem  TreatAsAtomicUnit=on  mask{slope=sigslopei, offset=0.5}
      mask help: Created by Han, Cheol
      mask Display: plot([10 15 20 25 30 35 40 45 50], [0 0.01 0.1 0.2 0.5 0.8 0.9 0.99 1])
  Out1 : Outport
  wires:
  ui/1 -> h(ui)/1(x), f(ui)/1(x)
  uj/1 -> f(uj)/1(x)
  f(ui)/1(y) -> Product/1
  f(uj)/1(y) -> Product/2
  Constant/1 -> Product/3
  Product/1 -> Sum/1
  Sum/1 -> Product1/2
  h(ui)/1(y) -> Product1/1
  Product1/1 -> Sum1/1
  beta/1 -> Sum1/2
  Sum1/1 -> 1_over_taus/1
  1_over_taus/1 -> Integrator/1
  Integrator/1 -> Switch1/1, Sum/2
  Sum2/1 -> Switch1/2
  Clock/1 -> Sum2/1
  Constant3/1 -> Sum2/2
  Switch1/1 -> beta/1, Out1/1
  Sij/1 -> Switch1/3

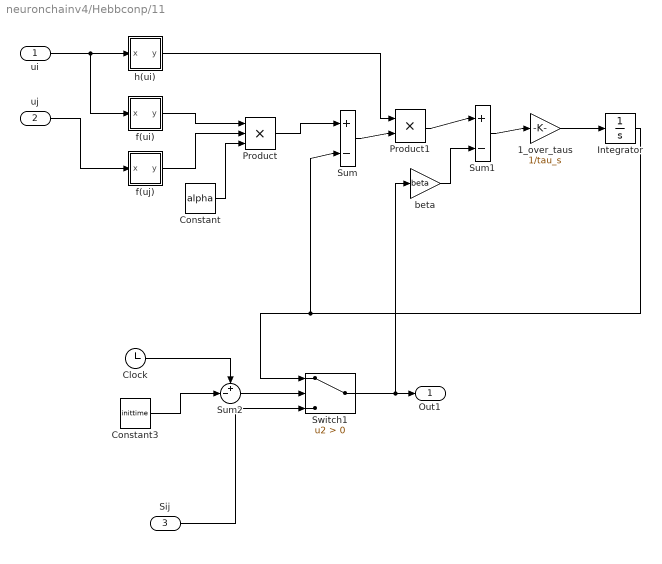
== system neuronchainv4/Hebbconp/11 ==
  ui : Inport
  uj : Inport  Port=2
  Sij : Inport  Port=3
  1_over_taus : Gain  Gain=1/tau_s
  Clock : Clock
      settings: Decimation=10
  Constant : Constant  Value=alpha
  Constant3 : Constant  Value=inittime
  Integrator : Integrator
  Product : Product  Inputs=3  RndMeth=Zero
  Product1 : Product  RndMeth=Zero
  Sum : Sum  Inputs=|+-
  Sum1 : Sum  Inputs=|+-
  Sum2 : Sum  Inputs=+-|
  Switch1 : Switch  Criteria=u2 > Threshold
  beta : Gain  Gain=beta
  f(ui) : Subsystem  TreatAsAtomicUnit=on  mask{slope=sigslopef, offset=0.5}
      mask help: Created by Han, Cheol
      mask Display: plot([10 15 20 25 30 35 40 45 50], [0 0.01 0.1 0.2 0.5 0.8 0.9 0.99 1])
  f(uj) : Subsystem  TreatAsAtomicUnit=on  mask{slope=sigslopef, offset=0.5}
      mask help: Created by Han, Cheol
      mask Display: plot([10 15 20 25 30 35 40 45 50], [0 0.01 0.1 0.2 0.5 0.8 0.9 0.99 1])
  h(ui) : Subsystem  TreatAsAtomicUnit=on  mask{slope=sigslopei, offset=0.5}
      mask help: Created by Han, Cheol
      mask Display: plot([10 15 20 25 30 35 40 45 50], [0 0.01 0.1 0.2 0.5 0.8 0.9 0.99 1])
  Out1 : Outport
  wires:
  ui/1 -> h(ui)/1(x), f(ui)/1(x)
  uj/1 -> f(uj)/1(x)
  f(ui)/1(y) -> Product/1
  f(uj)/1(y) -> Product/2
  Constant/1 -> Product/3
  Product/1 -> Sum/1
  Sum/1 -> Product1/2
  h(ui)/1(y) -> Product1/1
  Product1/1 -> Sum1/1
  beta/1 -> Sum1/2
  Sum1/1 -> 1_over_taus/1
  1_over_taus/1 -> Integrator/1
  Integrator/1 -> Switch1/1, Sum/2
  Sum2/1 -> Switch1/2
  Clock/1 -> Sum2/1
  Constant3/1 -> Sum2/2
  Switch1/1 -> beta/1, Out1/1
  Sij/1 -> Switch1/3

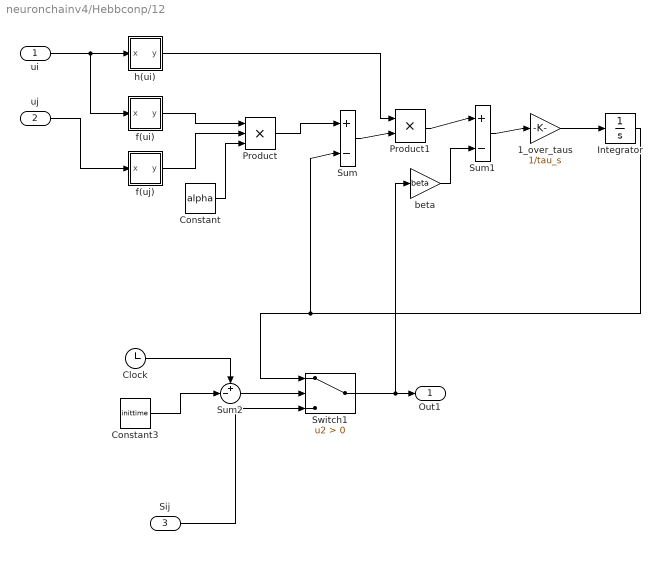
== system neuronchainv4/Hebbconp/12 ==
  ui : Inport
  uj : Inport  Port=2
  Sij : Inport  Port=3
  1_over_taus : Gain  Gain=1/tau_s
  Clock : Clock
      settings: Decimation=10
  Constant : Constant  Value=alpha
  Constant3 : Constant  Value=inittime
  Integrator : Integrator
  Product : Product  Inputs=3  RndMeth=Zero
  Product1 : Product  RndMeth=Zero
  Sum : Sum  Inputs=|+-
  Sum1 : Sum  Inputs=|+-
  Sum2 : Sum  Inputs=+-|
  Switch1 : Switch  Criteria=u2 > Threshold
  beta : Gain  Gain=beta
  f(ui) : Subsystem  TreatAsAtomicUnit=on  mask{slope=sigslopef, offset=0.5}
      mask help: Created by Han, Cheol
      mask Display: plot([10 15 20 25 30 35 40 45 50], [0 0.01 0.1 0.2 0.5 0.8 0.9 0.99 1])
  f(uj) : Subsystem  TreatAsAtomicUnit=on  mask{slope=sigslopef, offset=0.5}
      mask help: Created by Han, Cheol
      mask Display: plot([10 15 20 25 30 35 40 45 50], [0 0.01 0.1 0.2 0.5 0.8 0.9 0.99 1])
  h(ui) : Subsystem  TreatAsAtomicUnit=on  mask{slope=sigslopei, offset=0.5}
      mask help: Created by Han, Cheol
      mask Display: plot([10 15 20 25 30 35 40 45 50], [0 0.01 0.1 0.2 0.5 0.8 0.9 0.99 1])
  Out1 : Outport
  wires:
  ui/1 -> h(ui)/1(x), f(ui)/1(x)
  uj/1 -> f(uj)/1(x)
  f(ui)/1(y) -> Product/1
  f(uj)/1(y) -> Product/2
  Constant/1 -> Product/3
  Product/1 -> Sum/1
  Sum/1 -> Product1/2
  h(ui)/1(y) -> Product1/1
  Product1/1 -> Sum1/1
  beta/1 -> Sum1/2
  Sum1/1 -> 1_over_taus/1
  1_over_taus/1 -> Integrator/1
  Integrator/1 -> Switch1/1, Sum/2
  Sum2/1 -> Switch1/2
  Clock/1 -> Sum2/1
  Constant3/1 -> Sum2/2
  Switch1/1 -> beta/1, Out1/1
  Sij/1 -> Switch1/3

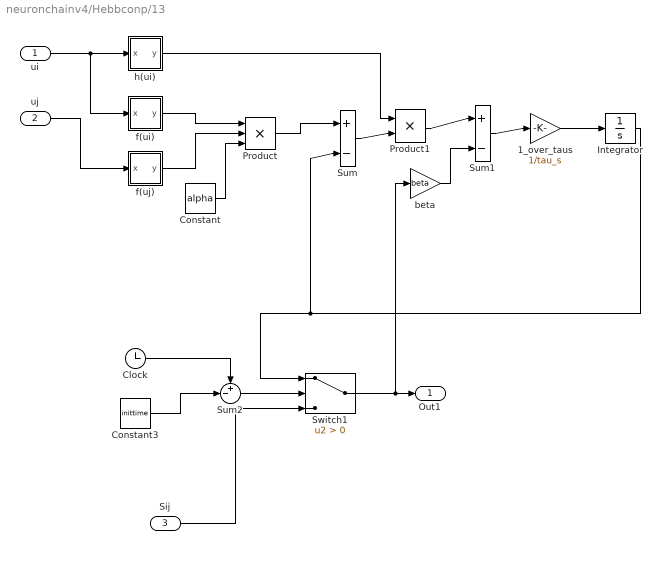
== system neuronchainv4/Hebbconp/13 ==
  ui : Inport
  uj : Inport  Port=2
  Sij : Inport  Port=3
  1_over_taus : Gain  Gain=1/tau_s
  Clock : Clock
      settings: Decimation=10
  Constant : Constant  Value=alpha
  Constant3 : Constant  Value=inittime
  Integrator : Integrator
  Product : Product  Inputs=3  RndMeth=Zero
  Product1 : Product  RndMeth=Zero
  Sum : Sum  Inputs=|+-
  Sum1 : Sum  Inputs=|+-
  Sum2 : Sum  Inputs=+-|
  Switch1 : Switch  Criteria=u2 > Threshold
  beta : Gain  Gain=beta
  f(ui) : Subsystem  TreatAsAtomicUnit=on  mask{slope=sigslopef, offset=0.5}
      mask help: Created by Han, Cheol
      mask Display: plot([10 15 20 25 30 35 40 45 50], [0 0.01 0.1 0.2 0.5 0.8 0.9 0.99 1])
  f(uj) : Subsystem  TreatAsAtomicUnit=on  mask{slope=sigslopef, offset=0.5}
      mask help: Created by Han, Cheol
      mask Display: plot([10 15 20 25 30 35 40 45 50], [0 0.01 0.1 0.2 0.5 0.8 0.9 0.99 1])
  h(ui) : Subsystem  TreatAsAtomicUnit=on  mask{slope=sigslopei, offset=0.5}
      mask help: Created by Han, Cheol
      mask Display: plot([10 15 20 25 30 35 40 45 50], [0 0.01 0.1 0.2 0.5 0.8 0.9 0.99 1])
  Out1 : Outport
  wires:
  ui/1 -> h(ui)/1(x), f(ui)/1(x)
  uj/1 -> f(uj)/1(x)
  f(ui)/1(y) -> Product/1
  f(uj)/1(y) -> Product/2
  Constant/1 -> Product/3
  Product/1 -> Sum/1
  Sum/1 -> Product1/2
  h(ui)/1(y) -> Product1/1
  Product1/1 -> Sum1/1
  beta/1 -> Sum1/2
  Sum1/1 -> 1_over_taus/1
  1_over_taus/1 -> Integrator/1
  Integrator/1 -> Switch1/1, Sum/2
  Sum2/1 -> Switch1/2
  Clock/1 -> Sum2/1
  Constant3/1 -> Sum2/2
  Switch1/1 -> beta/1, Out1/1
  Sij/1 -> Switch1/3

== system neuronchainv4/Hebbconp/14 ==
  ui : Inport
  uj : Inport  Port=2
  Sij : Inport  Port=3
  1_over_taus : Gain  Gain=1/tau_s
  Clock : Clock
      settings: Decimation=10
  Constant : Constant  Value=alpha
  Constant3 : Constant  Value=inittime
  Integrator : Integrator
  Product : Product  Inputs=3  RndMeth=Zero
  Product1 : Product  RndMeth=Zero
  Sum : Sum  Inputs=|+-
  Sum1 : Sum  Inputs=|+-
  Sum2 : Sum  Inputs=+-|
  Switch1 : Switch  Criteria=u2 > Threshold
  beta : Gain  Gain=beta
  f(ui) : Subsystem  TreatAsAtomicUnit=on  mask{slope=sigslopef, offset=0.5}
      mask help: Created by Han, Cheol
      mask Display: plot([10 15 20 25 30 35 40 45 50], [0 0.01 0.1 0.2 0.5 0.8 0.9 0.99 1])
  f(uj) : Subsystem  TreatAsAtomicUnit=on  mask{slope=sigslopef, offset=0.5}
      mask help: Created by Han, Cheol
      mask Display: plot([10 15 20 25 30 35 40 45 50], [0 0.01 0.1 0.2 0.5 0.8 0.9 0.99 1])
  h(ui) : Subsystem  TreatAsAtomicUnit=on  mask{slope=sigslopei, offset=0.5}
      mask help: Created by Han, Cheol
      mask Display: plot([10 15 20 25 30 35 40 45 50], [0 0.01 0.1 0.2 0.5 0.8 0.9 0.99 1])
  Out1 : Outport
  wires:
  ui/1 -> h(ui)/1(x), f(ui)/1(x)
  uj/1 -> f(uj)/1(x)
  f(ui)/1(y) -> Product/1
  f(uj)/1(y) -> Product/2
  Constant/1 -> Product/3
  Product/1 -> Sum/1
  Sum/1 -> Product1/2
  h(ui)/1(y) -> Product1/1
  Product1/1 -> Sum1/1
  beta/1 -> Sum1/2
  Sum1/1 -> 1_over_taus/1
  1_over_taus/1 -> Integrator/1
  Integrator/1 -> Switch1/1, Sum/2
  Sum2/1 -> Switch1/2
  Clock/1 -> Sum2/1
  Constant3/1 -> Sum2/2
  Switch1/1 -> beta/1, Out1/1
  Sij/1 -> Switch1/3

== system neuronchainv4/Hebbconp/15 ==
  ui : Inport
  uj : Inport  Port=2
  Sij : Inport  Port=3
  1_over_taus : Gain  Gain=1/tau_s
  Clock : Clock
      settings: Decimation=10
  Constant : Constant  Value=alpha
  Constant3 : Constant  Value=inittime
  Integrator : Integrator
  Product : Product  Inputs=3  RndMeth=Zero
  Product1 : Product  RndMeth=Zero
  Sum : Sum  Inputs=|+-
  Sum1 : Sum  Inputs=|+-
  Sum2 : Sum  Inputs=+-|
  Switch1 : Switch  Criteria=u2 > Threshold
  beta : Gain  Gain=beta
  f(ui) : Subsystem  TreatAsAtomicUnit=on  mask{slope=sigslopef, offset=0.5}
      mask help: Created by Han, Cheol
      mask Display: plot([10 15 20 25 30 35 40 45 50], [0 0.01 0.1 0.2 0.5 0.8 0.9 0.99 1])
  f(uj) : Subsystem  TreatAsAtomicUnit=on  mask{slope=sigslopef, offset=0.5}
      mask help: Created by Han, Cheol
      mask Display: plot([10 15 20 25 30 35 40 45 50], [0 0.01 0.1 0.2 0.5 0.8 0.9 0.99 1])
  h(ui) : Subsystem  TreatAsAtomicUnit=on  mask{slope=sigslopei, offset=0.5}
      mask help: Created by Han, Cheol
      mask Display: plot([10 15 20 25 30 35 40 45 50], [0 0.01 0.1 0.2 0.5 0.8 0.9 0.99 1])
  Out1 : Outport
  wires:
  ui/1 -> h(ui)/1(x), f(ui)/1(x)
  uj/1 -> f(uj)/1(x)
  f(ui)/1(y) -> Product/1
  f(uj)/1(y) -> Product/2
  Constant/1 -> Product/3
  Product/1 -> Sum/1
  Sum/1 -> Product1/2
  h(ui)/1(y) -> Product1/1
  Product1/1 -> Sum1/1
  beta/1 -> Sum1/2
  Sum1/1 -> 1_over_taus/1
  1_over_taus/1 -> Integrator/1
  Integrator/1 -> Switch1/1, Sum/2
  Sum2/1 -> Switch1/2
  Clock/1 -> Sum2/1
  Constant3/1 -> Sum2/2
  Switch1/1 -> beta/1, Out1/1
  Sij/1 -> Switch1/3

== system neuronchainv4/Hebbconp/21 ==
  ui : Inport
  uj : Inport  Port=2
  Sij : Inport  Port=3
  1_over_taus : Gain  Gain=1/tau_s
  Clock : Clock
      settings: Decimation=10
  Constant : Constant  Value=alpha
  Constant3 : Constant  Value=inittime
  Integrator : Integrator
  Product : Product  Inputs=3  RndMeth=Zero
  Product1 : Product  RndMeth=Zero
  Sum : Sum  Inputs=|+-
  Sum1 : Sum  Inputs=|+-
  Sum2 : Sum  Inputs=+-|
  Switch1 : Switch  Criteria=u2 > Threshold
  beta : Gain  Gain=beta
  f(ui) : Subsystem  TreatAsAtomicUnit=on  mask{slope=sigslopef, offset=0.5}
      mask help: Created by Han, Cheol
      mask Display: plot([10 15 20 25 30 35 40 45 50], [0 0.01 0.1 0.2 0.5 0.8 0.9 0.99 1])
  f(uj) : Subsystem  TreatAsAtomicUnit=on  mask{slope=sigslopef, offset=0.5}
      mask help: Created by Han, Cheol
      mask Display: plot([10 15 20 25 30 35 40 45 50], [0 0.01 0.1 0.2 0.5 0.8 0.9 0.99 1])
  h(ui) : Subsystem  TreatAsAtomicUnit=on  mask{slope=sigslopei, offset=0.5}
      mask help: Created by Han, Cheol
      mask Display: plot([10 15 20 25 30 35 40 45 50], [0 0.01 0.1 0.2 0.5 0.8 0.9 0.99 1])
  Out1 : Outport
  wires:
  ui/1 -> h(ui)/1(x), f(ui)/1(x)
  uj/1 -> f(uj)/1(x)
  f(ui)/1(y) -> Product/1
  f(uj)/1(y) -> Product/2
  Constant/1 -> Product/3
  Product/1 -> Sum/1
  Sum/1 -> Product1/2
  h(ui)/1(y) -> Product1/1
  Product1/1 -> Sum1/1
  beta/1 -> Sum1/2
  Sum1/1 -> 1_over_taus/1
  1_over_taus/1 -> Integrator/1
  Integrator/1 -> Switch1/1, Sum/2
  Sum2/1 -> Switch1/2
  Clock/1 -> Sum2/1
  Constant3/1 -> Sum2/2
  Switch1/1 -> beta/1, Out1/1
  Sij/1 -> Switch1/3

== system neuronchainv4/Hebbconp/22 ==
  ui : Inport
  uj : Inport  Port=2
  Sij : Inport  Port=3
  1_over_taus : Gain  Gain=1/tau_s
  Clock : Clock
      settings: Decimation=10
  Constant : Constant  Value=alpha
  Constant3 : Constant  Value=inittime
  Integrator : Integrator
  Product : Product  Inputs=3  RndMeth=Zero
  Product1 : Product  RndMeth=Zero
  Sum : Sum  Inputs=|+-
  Sum1 : Sum  Inputs=|+-
  Sum2 : Sum  Inputs=+-|
  Switch1 : Switch  Criteria=u2 > Threshold
  beta : Gain  Gain=beta
  f(ui) : Subsystem  TreatAsAtomicUnit=on  mask{slope=sigslopef, offset=0.5}
      mask help: Created by Han, Cheol
      mask Display: plot([10 15 20 25 30 35 40 45 50], [0 0.01 0.1 0.2 0.5 0.8 0.9 0.99 1])
  f(uj) : Subsystem  TreatAsAtomicUnit=on  mask{slope=sigslopef, offset=0.5}
      mask help: Created by Han, Cheol
      mask Display: plot([10 15 20 25 30 35 40 45 50], [0 0.01 0.1 0.2 0.5 0.8 0.9 0.99 1])
  h(ui) : Subsystem  TreatAsAtomicUnit=on  mask{slope=sigslopei, offset=0.5}
      mask help: Created by Han, Cheol
      mask Display: plot([10 15 20 25 30 35 40 45 50], [0 0.01 0.1 0.2 0.5 0.8 0.9 0.99 1])
  Out1 : Outport
  wires:
  ui/1 -> h(ui)/1(x), f(ui)/1(x)
  uj/1 -> f(uj)/1(x)
  f(ui)/1(y) -> Product/1
  f(uj)/1(y) -> Product/2
  Constant/1 -> Product/3
  Product/1 -> Sum/1
  Sum/1 -> Product1/2
  h(ui)/1(y) -> Product1/1
  Product1/1 -> Sum1/1
  beta/1 -> Sum1/2
  Sum1/1 -> 1_over_taus/1
  1_over_taus/1 -> Integrator/1
  Integrator/1 -> Switch1/1, Sum/2
  Sum2/1 -> Switch1/2
  Clock/1 -> Sum2/1
  Constant3/1 -> Sum2/2
  Switch1/1 -> beta/1, Out1/1
  Sij/1 -> Switch1/3

== system neuronchainv4/Hebbconp/23 ==
  ui : Inport
  uj : Inport  Port=2
  Sij : Inport  Port=3
  1_over_taus : Gain  Gain=1/tau_s
  Clock : Clock
      settings: Decimation=10
  Constant : Constant  Value=alpha
  Constant3 : Constant  Value=inittime
  Integrator : Integrator
  Product : Product  Inputs=3  RndMeth=Zero
  Product1 : Product  RndMeth=Zero
  Sum : Sum  Inputs=|+-
  Sum1 : Sum  Inputs=|+-
  Sum2 : Sum  Inputs=+-|
  Switch1 : Switch  Criteria=u2 > Threshold
  beta : Gain  Gain=beta
  f(ui) : Subsystem  TreatAsAtomicUnit=on  mask{slope=sigslopef, offset=0.5}
      mask help: Created by Han, Cheol
      mask Display: plot([10 15 20 25 30 35 40 45 50], [0 0.01 0.1 0.2 0.5 0.8 0.9 0.99 1])
  f(uj) : Subsystem  TreatAsAtomicUnit=on  mask{slope=sigslopef, offset=0.5}
      mask help: Created by Han, Cheol
      mask Display: plot([10 15 20 25 30 35 40 45 50], [0 0.01 0.1 0.2 0.5 0.8 0.9 0.99 1])
  h(ui) : Subsystem  TreatAsAtomicUnit=on  mask{slope=sigslopei, offset=0.5}
      mask help: Created by Han, Cheol
      mask Display: plot([10 15 20 25 30 35 40 45 50], [0 0.01 0.1 0.2 0.5 0.8 0.9 0.99 1])
  Out1 : Outport
  wires:
  ui/1 -> h(ui)/1(x), f(ui)/1(x)
  uj/1 -> f(uj)/1(x)
  f(ui)/1(y) -> Product/1
  f(uj)/1(y) -> Product/2
  Constant/1 -> Product/3
  Product/1 -> Sum/1
  Sum/1 -> Product1/2
  h(ui)/1(y) -> Product1/1
  Product1/1 -> Sum1/1
  beta/1 -> Sum1/2
  Sum1/1 -> 1_over_taus/1
  1_over_taus/1 -> Integrator/1
  Integrator/1 -> Switch1/1, Sum/2
  Sum2/1 -> Switch1/2
  Clock/1 -> Sum2/1
  Constant3/1 -> Sum2/2
  Switch1/1 -> beta/1, Out1/1
  Sij/1 -> Switch1/3

== system neuronchainv4/Hebbconp/24 ==
  ui : Inport
  uj : Inport  Port=2
  Sij : Inport  Port=3
  1_over_taus : Gain  Gain=1/tau_s
  Clock : Clock
      settings: Decimation=10
  Constant : Constant  Value=alpha
  Constant3 : Constant  Value=inittime
  Integrator : Integrator
  Product : Product  Inputs=3  RndMeth=Zero
  Product1 : Product  RndMeth=Zero
  Sum : Sum  Inputs=|+-
  Sum1 : Sum  Inputs=|+-
  Sum2 : Sum  Inputs=+-|
  Switch1 : Switch  Criteria=u2 > Threshold
  beta : Gain  Gain=beta
  f(ui) : Subsystem  TreatAsAtomicUnit=on  mask{slope=sigslopef, offset=0.5}
      mask help: Created by Han, Cheol
      mask Display: plot([10 15 20 25 30 35 40 45 50], [0 0.01 0.1 0.2 0.5 0.8 0.9 0.99 1])
  f(uj) : Subsystem  TreatAsAtomicUnit=on  mask{slope=sigslopef, offset=0.5}
      mask help: Created by Han, Cheol
      mask Display: plot([10 15 20 25 30 35 40 45 50], [0 0.01 0.1 0.2 0.5 0.8 0.9 0.99 1])
  h(ui) : Subsystem  TreatAsAtomicUnit=on  mask{slope=sigslopei, offset=0.5}
      mask help: Created by Han, Cheol
      mask Display: plot([10 15 20 25 30 35 40 45 50], [0 0.01 0.1 0.2 0.5 0.8 0.9 0.99 1])
  Out1 : Outport
  wires:
  ui/1 -> h(ui)/1(x), f(ui)/1(x)
  uj/1 -> f(uj)/1(x)
  f(ui)/1(y) -> Product/1
  f(uj)/1(y) -> Product/2
  Constant/1 -> Product/3
  Product/1 -> Sum/1
  Sum/1 -> Product1/2
  h(ui)/1(y) -> Product1/1
  Product1/1 -> Sum1/1
  beta/1 -> Sum1/2
  Sum1/1 -> 1_over_taus/1
  1_over_taus/1 -> Integrator/1
  Integrator/1 -> Switch1/1, Sum/2
  Sum2/1 -> Switch1/2
  Clock/1 -> Sum2/1
  Constant3/1 -> Sum2/2
  Switch1/1 -> beta/1, Out1/1
  Sij/1 -> Switch1/3

== system neuronchainv4/Hebbconp/25 ==
  ui : Inport
  uj : Inport  Port=2
  Sij : Inport  Port=3
  1_over_taus : Gain  Gain=1/tau_s
  Clock : Clock
      settings: Decimation=10
  Constant : Constant  Value=alpha
  Constant3 : Constant  Value=inittime
  Integrator : Integrator
  Product : Product  Inputs=3  RndMeth=Zero
  Product1 : Product  RndMeth=Zero
  Sum : Sum  Inputs=|+-
  Sum1 : Sum  Inputs=|+-
  Sum2 : Sum  Inputs=+-|
  Switch1 : Switch  Criteria=u2 > Threshold
  beta : Gain  Gain=beta
  f(ui) : Subsystem  TreatAsAtomicUnit=on  mask{slope=sigslopef, offset=0.5}
      mask help: Created by Han, Cheol
      mask Display: plot([10 15 20 25 30 35 40 45 50], [0 0.01 0.1 0.2 0.5 0.8 0.9 0.99 1])
  f(uj) : Subsystem  TreatAsAtomicUnit=on  mask{slope=sigslopef, offset=0.5}
      mask help: Created by Han, Cheol
      mask Display: plot([10 15 20 25 30 35 40 45 50], [0 0.01 0.1 0.2 0.5 0.8 0.9 0.99 1])
  h(ui) : Subsystem  TreatAsAtomicUnit=on  mask{slope=sigslopei, offset=0.5}
      mask help: Created by Han, Cheol
      mask Display: plot([10 15 20 25 30 35 40 45 50], [0 0.01 0.1 0.2 0.5 0.8 0.9 0.99 1])
  Out1 : Outport
  wires:
  ui/1 -> h(ui)/1(x), f(ui)/1(x)
  uj/1 -> f(uj)/1(x)
  f(ui)/1(y) -> Product/1
  f(uj)/1(y) -> Product/2
  Constant/1 -> Product/3
  Product/1 -> Sum/1
  Sum/1 -> Product1/2
  h(ui)/1(y) -> Product1/1
  Product1/1 -> Sum1/1
  beta/1 -> Sum1/2
  Sum1/1 -> 1_over_taus/1
  1_over_taus/1 -> Integrator/1
  Integrator/1 -> Switch1/1, Sum/2
  Sum2/1 -> Switch1/2
  Clock/1 -> Sum2/1
  Constant3/1 -> Sum2/2
  Switch1/1 -> beta/1, Out1/1
  Sij/1 -> Switch1/3

== system neuronchainv4/Hebbconp/3 ==
  ui : Inport
  uj : Inport  Port=2
  Sij : Inport  Port=3
  1_over_taus : Gain  Gain=1/tau_s
  Clock : Clock
      settings: Decimation=10
  Constant : Constant  Value=alpha
  Constant3 : Constant  Value=inittime
  Integrator : Integrator
  Product : Product  Inputs=3  RndMeth=Zero
  Product1 : Product  RndMeth=Zero
  Sum : Sum  Inputs=|+-
  Sum1 : Sum  Inputs=|+-
  Sum2 : Sum  Inputs=+-|
  Switch1 : Switch  Criteria=u2 > Threshold
  beta : Gain  Gain=beta
  f(ui) : Subsystem  TreatAsAtomicUnit=on  mask{slope=sigslopef, offset=0.5}
      mask help: Created by Han, Cheol
      mask Display: plot([10 15 20 25 30 35 40 45 50], [0 0.01 0.1 0.2 0.5 0.8 0.9 0.99 1])
  f(uj) : Subsystem  TreatAsAtomicUnit=on  mask{slope=sigslopef, offset=0.5}
      mask help: Created by Han, Cheol
      mask Display: plot([10 15 20 25 30 35 40 45 50], [0 0.01 0.1 0.2 0.5 0.8 0.9 0.99 1])
  h(ui) : Subsystem  TreatAsAtomicUnit=on  mask{slope=sigslopei, offset=0.5}
      mask help: Created by Han, Cheol
      mask Display: plot([10 15 20 25 30 35 40 45 50], [0 0.01 0.1 0.2 0.5 0.8 0.9 0.99 1])
  Out1 : Outport
  wires:
  ui/1 -> h(ui)/1(x), f(ui)/1(x)
  uj/1 -> f(uj)/1(x)
  f(ui)/1(y) -> Product/1
  f(uj)/1(y) -> Product/2
  Constant/1 -> Product/3
  Product/1 -> Sum/1
  Sum/1 -> Product1/2
  h(ui)/1(y) -> Product1/1
  Product1/1 -> Sum1/1
  beta/1 -> Sum1/2
  Sum1/1 -> 1_over_taus/1
  1_over_taus/1 -> Integrator/1
  Integrator/1 -> Switch1/1, Sum/2
  Sum2/1 -> Switch1/2
  Clock/1 -> Sum2/1
  Constant3/1 -> Sum2/2
  Switch1/1 -> beta/1, Out1/1
  Sij/1 -> Switch1/3

== system neuronchainv4/Hebbconp/31 ==
  ui : Inport
  uj : Inport  Port=2
  Sij : Inport  Port=3
  1_over_taus : Gain  Gain=1/tau_s
  Clock : Clock
      settings: Decimation=10
  Constant : Constant  Value=alpha
  Constant3 : Constant  Value=inittime
  Integrator : Integrator
  Product : Product  Inputs=3  RndMeth=Zero
  Product1 : Product  RndMeth=Zero
  Sum : Sum  Inputs=|+-
  Sum1 : Sum  Inputs=|+-
  Sum2 : Sum  Inputs=+-|
  Switch1 : Switch  Criteria=u2 > Threshold
  beta : Gain  Gain=beta
  f(ui) : Subsystem  TreatAsAtomicUnit=on  mask{slope=sigslopef, offset=0.5}
      mask help: Created by Han, Cheol
      mask Display: plot([10 15 20 25 30 35 40 45 50], [0 0.01 0.1 0.2 0.5 0.8 0.9 0.99 1])
  f(uj) : Subsystem  TreatAsAtomicUnit=on  mask{slope=sigslopef, offset=0.5}
      mask help: Created by Han, Cheol
      mask Display: plot([10 15 20 25 30 35 40 45 50], [0 0.01 0.1 0.2 0.5 0.8 0.9 0.99 1])
  h(ui) : Subsystem  TreatAsAtomicUnit=on  mask{slope=sigslopei, offset=0.5}
      mask help: Created by Han, Cheol
      mask Display: plot([10 15 20 25 30 35 40 45 50], [0 0.01 0.1 0.2 0.5 0.8 0.9 0.99 1])
  Out1 : Outport
  wires:
  ui/1 -> h(ui)/1(x), f(ui)/1(x)
  uj/1 -> f(uj)/1(x)
  f(ui)/1(y) -> Product/1
  f(uj)/1(y) -> Product/2
  Constant/1 -> Product/3
  Product/1 -> Sum/1
  Sum/1 -> Product1/2
  h(ui)/1(y) -> Product1/1
  Product1/1 -> Sum1/1
  beta/1 -> Sum1/2
  Sum1/1 -> 1_over_taus/1
  1_over_taus/1 -> Integrator/1
  Integrator/1 -> Switch1/1, Sum/2
  Sum2/1 -> Switch1/2
  Clock/1 -> Sum2/1
  Constant3/1 -> Sum2/2
  Switch1/1 -> beta/1, Out1/1
  Sij/1 -> Switch1/3
